simulink model "SS_1029"  (R2014a)
settings: Solver=FixedStepDiscrete  StartTime=0.0  StopTime=5  FixedStep=0.0005  RelTol=1e-3
values from neighbouring files (symbols this model uses):
  APS_High_null = ecucoder_cal(APS_High_null)    [SS.m]
  APS_High_x = ecucoder_cal(APS_High_x)    [SS.m]
  APS_High_y = ecucoder_cal(APS_High_y)    [SS.m]
  APS_Low_null = ecucoder_cal(APS_Low_null)    [SS.m]
  APS_low_x = ecucoder_cal(APS_low_x)    [SS.m]
  APS_low_y = ecucoder_cal(APS_low_y)    [SS.m]
  BrakeSignal_cal = ecucoder_cal(BrakeSignal_cal)    [SS.m]
  CustomReduceFactor_cal = ecucoder_cal(CustomReduceFactor_cal)    [SS.m]
  Differential_cal = ecucoder_cal(Differential_cal)    [SS.m]
  LowSOCWarning_cal = ecucoder_cal(LowSOCWarning_cal)    [SS.m]
  MotorTemperatureHigh_cal = ecucoder_cal(MotorTemperatureHigh_cal)    [SS.m]
  MotorTemperatureLow_cal = ecucoder_cal(MotorTemperatureLow_cal)    [SS.m]
  OilPressure_x = ecucoder_cal(OilPressure_x)    [SS.m]
  OilPressure_y = ecucoder_cal(OilPressure_y)    [SS.m]
  PowerBias_cal = ecucoder_cal(PowerBias_cal)    [SS.m]
  SpeedLimitFactor_x = ecucoder_cal(SpeedLimitFactor_x)    [SS.m]
  SpeedLimitFactor_y = ecucoder_cal(SpeedLimitFactor_y)    [SS.m]
  TorqueLimitNegativ_cal = ecucoder_cal(TorqueLimitNegativ_cal)    [SS.m]
  TorqueLimitPositiv_cal = ecucoder_cal(TorqueLimitPositiv_cal)    [SS.m]
libraries: simulink x101, ec55xxlib x31
(part 2 of 3)

== system SS_1029/HardWare_Input/In1_Message/Function-Call Subsystem1 ==
  Enable : Inport
  CANMsg : Inport  Port=2
  function : TriggerPort  TriggerType=function-call
  Subsystem : Subsystem
  AMK_TempMotor : Outport
  AMK_TempInverter : Outport  Port=2
  wires:
  CANMsg/1 -> Subsystem/1(In1)
  Subsystem/1(AMK_TempMotor) -> AMK_TempMotor/1
  Subsystem/2(AMK_TempInverter) -> AMK_TempInverter/1
  Enable/1 -> Subsystem/Enable

== system SS_1029/HardWare_Input/In2_Message/Function-Call Subsystem ==
  Enable : Inport
  CANMsg : Inport  Port=2
  function : TriggerPort  TriggerType=function-call
  Subsystem1 : Subsystem
  AMK_ActuralVelocity : Outport
  AMK_ActuralTorque : Outport  Port=2
  AMK_bSystemReady : Outport  Port=3
  AMK_bError : Outport  Port=4
  AMK_bQuitDcOn : Outport  Port=5
  "AMK_bQuitInverterOn " : Outport  Port=6
  wires:
  CANMsg/1 -> Subsystem1/1(In1)
  Subsystem1/1(Out1) -> AMK_bSystemReady/1
  Subsystem1/2(Out2) -> AMK_bError/1
  Subsystem1/3(Out3) -> AMK_bQuitDcOn/1
  Subsystem1/4(Out4) -> "AMK_bQuitInverterOn "/1
  Subsystem1/5(Out5) -> AMK_ActuralVelocity/1
  Subsystem1/6(Out6) -> AMK_ActuralTorque/1
  Enable/1 -> Subsystem1/Enable

== system SS_1029/HardWare_Input/In2_Message/Function-Call Subsystem1 ==
  Enable : Inport
  CANMsg : Inport  Port=2
  function : TriggerPort  TriggerType=function-call
  Subsystem : Subsystem
  AMK_TempMotor : Outport
  AMK_TempInverter : Outport  Port=2
  wires:
  CANMsg/1 -> Subsystem/1(In1)
  Subsystem/1(AMK_TempMotor) -> AMK_TempMotor/1
  Subsystem/2(AMK_TempInverter) -> AMK_TempInverter/1
  Enable/1 -> Subsystem/Enable

== system SS_1029/HardWare_Input/In3_Message/Function-Call Subsystem ==
  Enable : Inport
  CANMsg : Inport  Port=2
  function : TriggerPort  TriggerType=function-call
  Subsystem1 : Subsystem
  AMK_ActuralVelocity : Outport
  AMK_ActuralTorque : Outport  Port=2
  AMK_bSystemReady : Outport  Port=3
  AMK_bError : Outport  Port=4
  AMK_bQuitDcOn : Outport  Port=5
  "AMK_bQuitInverterOn " : Outport  Port=6
  wires:
  CANMsg/1 -> Subsystem1/1(In1)
  Subsystem1/1(Out1) -> AMK_bSystemReady/1
  Subsystem1/2(Out2) -> AMK_bError/1
  Subsystem1/3(Out3) -> AMK_bQuitDcOn/1
  Subsystem1/4(Out4) -> "AMK_bQuitInverterOn "/1
  Subsystem1/5(Out5) -> AMK_ActuralVelocity/1
  Subsystem1/6(Out6) -> AMK_ActuralTorque/1
  Enable/1 -> Subsystem1/Enable

== system SS_1029/HardWare_Input/In3_Message/Function-Call Subsystem1 ==
  Enable : Inport
  CANMsg : Inport  Port=2
  function : TriggerPort  TriggerType=function-call
  Subsystem : Subsystem
  AMK_TempMotor : Outport
  AMK_TempInverter : Outport  Port=2
  wires:
  CANMsg/1 -> Subsystem/1(In1)
  Subsystem/1(AMK_TempMotor) -> AMK_TempMotor/1
  Subsystem/2(AMK_TempInverter) -> AMK_TempInverter/1
  Enable/1 -> Subsystem/Enable

== system SS_1029/HardWare_Input/In4_Message/Function-Call Subsystem ==
  Enable : Inport
  CANMsg : Inport  Port=2
  function : TriggerPort  TriggerType=function-call
  Subsystem1 : Subsystem
  AMK_ActuralVelocity : Outport
  AMK_ActuralTorque : Outport  Port=2
  AMK_bSystemReady : Outport  Port=3
  AMK_bError : Outport  Port=4
  AMK_bQuitDcOn : Outport  Port=5
  "AMK_bQuitInverterOn " : Outport  Port=6
  wires:
  CANMsg/1 -> Subsystem1/1(In1)
  Subsystem1/1(Out1) -> AMK_bSystemReady/1
  Subsystem1/2(Out2) -> AMK_bError/1
  Subsystem1/3(Out3) -> AMK_bQuitDcOn/1
  Subsystem1/4(Out4) -> "AMK_bQuitInverterOn "/1
  Subsystem1/5(Out5) -> AMK_ActuralVelocity/1
  Subsystem1/6(Out6) -> AMK_ActuralTorque/1
  Enable/1 -> Subsystem1/Enable

== system SS_1029/HardWare_Input/In4_Message/Function-Call Subsystem1 ==
  Enable : Inport
  CANMsg : Inport  Port=2
  function : TriggerPort  TriggerType=function-call
  Subsystem : Subsystem
  AMK_TempMotor : Outport
  AMK_TempInverter : Outport  Port=2
  wires:
  CANMsg/1 -> Subsystem/1(In1)
  Subsystem/1(AMK_TempMotor) -> AMK_TempMotor/1
  Subsystem/2(AMK_TempInverter) -> AMK_TempInverter/1
  Enable/1 -> Subsystem/Enable

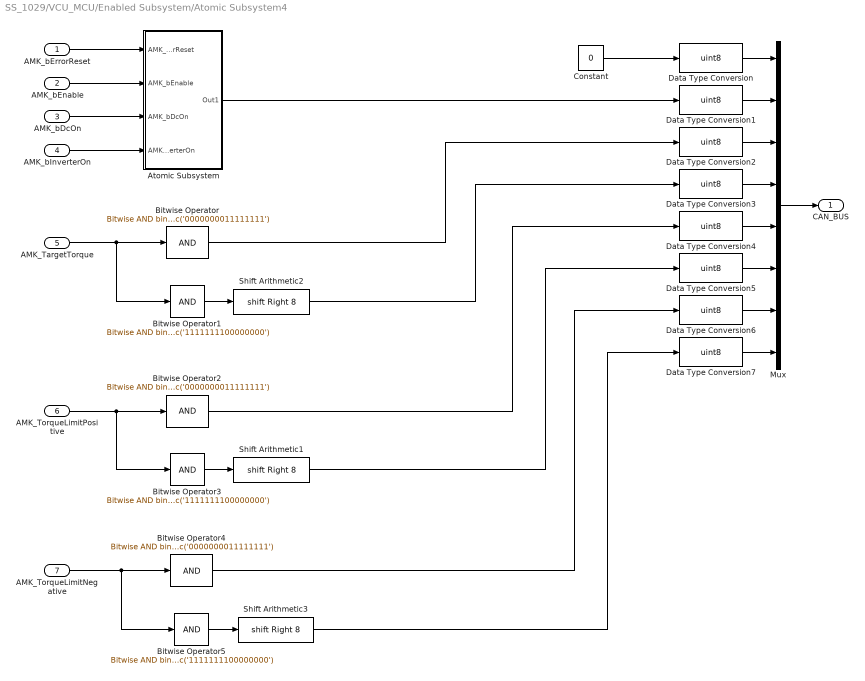
== system SS_1029/VCU_MCU/Enabled Subsystem/Atomic Subsystem4 ==
  AMK_bErrorReset : Inport
  AMK_bEnable : Inport  Port=2
  AMK_bDcOn : Inport  Port=3
  AMK_bInverterOn : Inport  Port=4
  AMK_TargetTorque : Inport  Port=5
  AMK_TorqueLimitPositive : Inport  Port=6
  AMK_TorqueLimitNegative : Inport  Port=7
  Atomic Subsystem : Subsystem  TreatAsAtomicUnit=on
  Bitwise Operator : simulink/Logic and Bit Operations/Bitwise Operator  logicop=AND  UseBitMask=on  BitMask=bin2dec('0000000011111111')  BitMaskRealWorld=Stored Integer
  Bitwise Operator1 : simulink/Logic and Bit Operations/Bitwise Operator  logicop=AND  UseBitMask=on  BitMask=bin2dec('1111111100000000')  BitMaskRealWorld=Stored Integer
  Bitwise Operator2 : simulink/Logic and Bit Operations/Bitwise Operator  logicop=AND  UseBitMask=on  BitMask=bin2dec('0000000011111111')  BitMaskRealWorld=Stored Integer
  Bitwise Operator3 : simulink/Logic and Bit Operations/Bitwise Operator  logicop=AND  UseBitMask=on  BitMask=bin2dec('1111111100000000')  BitMaskRealWorld=Stored Integer
  Bitwise Operator4 : simulink/Logic and Bit Operations/Bitwise Operator  logicop=AND  UseBitMask=on  BitMask=bin2dec('0000000011111111')  BitMaskRealWorld=Stored Integer
  Bitwise Operator5 : simulink/Logic and Bit Operations/Bitwise Operator  logicop=AND  UseBitMask=on  BitMask=bin2dec('1111111100000000')  BitMaskRealWorld=Stored Integer
  Constant : Constant  Value=0  OutDataTypeStr=uint8  SampleTime=-1
  Data Type Conversion{,1..7} (8 alike) : DataTypeConversion  OutDataTypeStr=uint8
  Mux : Mux  Inputs=8
  Shift Arithmetic1 : ArithShift  BitShiftNumber=8  BitShiftDirection=Right
  Shift Arithmetic2 : ArithShift  BitShiftNumber=8  BitShiftDirection=Right
  Shift Arithmetic3 : ArithShift  BitShiftNumber=8  BitShiftDirection=Right
  CAN_BUS : Outport
  wires:
  Mux/1 -> CAN_BUS/1
  Data Type Conversion/1 -> Mux/1
  Data Type Conversion1/1 -> Mux/2
  Data Type Conversion2/1 -> Mux/3
  Data Type Conversion3/1 -> Mux/4
  Data Type Conversion4/1 -> Mux/5
  Data Type Conversion5/1 -> Mux/6
  Data Type Conversion6/1 -> Mux/7
  Data Type Conversion7/1 -> Mux/8
  Constant/1 -> Data Type Conversion/1
  AMK_bErrorReset/1 -> Atomic Subsystem/1(AMK_bErrorReset)
  AMK_bEnable/1 -> Atomic Subsystem/2(AMK_bEnable)
  AMK_bDcOn/1 -> Atomic Subsystem/3(AMK_bDcOn)
  AMK_bInverterOn/1 -> Atomic Subsystem/4(AMK_bInverterOn)
  Atomic Subsystem/1(Out1) -> Data Type Conversion1/1
  AMK_TargetTorque/1 -> Bitwise Operator1/1, Bitwise Operator/1
  Bitwise Operator/1 -> Data Type Conversion2/1
  Bitwise Operator1/1 -> Shift Arithmetic2/1
  Shift Arithmetic2/1 -> Data Type Conversion3/1
  AMK_TorqueLimitPositive/1 -> Bitwise Operator3/1, Bitwise Operator2/1
  Bitwise Operator3/1 -> Shift Arithmetic1/1
  Bitwise Operator2/1 -> Data Type Conversion4/1
  Shift Arithmetic1/1 -> Data Type Conversion5/1
  AMK_TorqueLimitNegative/1 -> Bitwise Operator5/1, Bitwise Operator4/1
  Bitwise Operator5/1 -> Shift Arithmetic3/1
  Bitwise Operator4/1 -> Data Type Conversion6/1
  Shift Arithmetic3/1 -> Data Type Conversion7/1

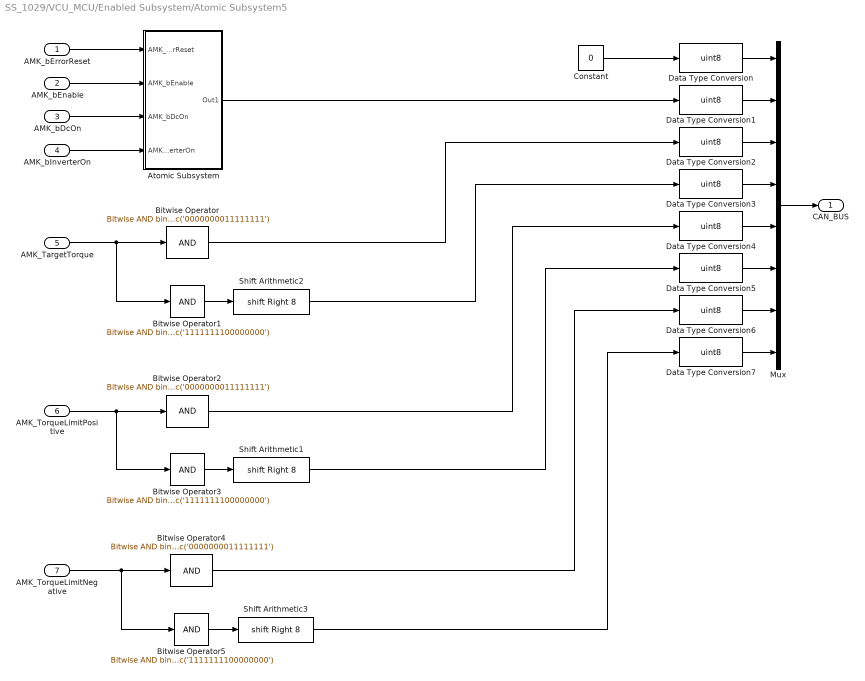
== system SS_1029/VCU_MCU/Enabled Subsystem/Atomic Subsystem5 ==
  AMK_bErrorReset : Inport
  AMK_bEnable : Inport  Port=2
  AMK_bDcOn : Inport  Port=3
  AMK_bInverterOn : Inport  Port=4
  AMK_TargetTorque : Inport  Port=5
  AMK_TorqueLimitPositive : Inport  Port=6
  AMK_TorqueLimitNegative : Inport  Port=7
  Atomic Subsystem : Subsystem  TreatAsAtomicUnit=on
  Bitwise Operator : simulink/Logic and Bit Operations/Bitwise Operator  logicop=AND  UseBitMask=on  BitMask=bin2dec('0000000011111111')  BitMaskRealWorld=Stored Integer
  Bitwise Operator1 : simulink/Logic and Bit Operations/Bitwise Operator  logicop=AND  UseBitMask=on  BitMask=bin2dec('1111111100000000')  BitMaskRealWorld=Stored Integer
  Bitwise Operator2 : simulink/Logic and Bit Operations/Bitwise Operator  logicop=AND  UseBitMask=on  BitMask=bin2dec('0000000011111111')  BitMaskRealWorld=Stored Integer
  Bitwise Operator3 : simulink/Logic and Bit Operations/Bitwise Operator  logicop=AND  UseBitMask=on  BitMask=bin2dec('1111111100000000')  BitMaskRealWorld=Stored Integer
  Bitwise Operator4 : simulink/Logic and Bit Operations/Bitwise Operator  logicop=AND  UseBitMask=on  BitMask=bin2dec('0000000011111111')  BitMaskRealWorld=Stored Integer
  Bitwise Operator5 : simulink/Logic and Bit Operations/Bitwise Operator  logicop=AND  UseBitMask=on  BitMask=bin2dec('1111111100000000')  BitMaskRealWorld=Stored Integer
  Constant : Constant  Value=0  OutDataTypeStr=uint8  SampleTime=-1
  Data Type Conversion{,1..7} (8 alike) : DataTypeConversion  OutDataTypeStr=uint8
  Mux : Mux  Inputs=8
  Shift Arithmetic1 : ArithShift  BitShiftNumber=8  BitShiftDirection=Right
  Shift Arithmetic2 : ArithShift  BitShiftNumber=8  BitShiftDirection=Right
  Shift Arithmetic3 : ArithShift  BitShiftNumber=8  BitShiftDirection=Right
  CAN_BUS : Outport
  wires:
  Mux/1 -> CAN_BUS/1
  Data Type Conversion/1 -> Mux/1
  Data Type Conversion1/1 -> Mux/2
  Data Type Conversion2/1 -> Mux/3
  Data Type Conversion3/1 -> Mux/4
  Data Type Conversion4/1 -> Mux/5
  Data Type Conversion5/1 -> Mux/6
  Data Type Conversion6/1 -> Mux/7
  Data Type Conversion7/1 -> Mux/8
  Constant/1 -> Data Type Conversion/1
  AMK_bErrorReset/1 -> Atomic Subsystem/1(AMK_bErrorReset)
  AMK_bEnable/1 -> Atomic Subsystem/2(AMK_bEnable)
  AMK_bDcOn/1 -> Atomic Subsystem/3(AMK_bDcOn)
  AMK_bInverterOn/1 -> Atomic Subsystem/4(AMK_bInverterOn)
  Atomic Subsystem/1(Out1) -> Data Type Conversion1/1
  AMK_TargetTorque/1 -> Bitwise Operator1/1, Bitwise Operator/1
  Bitwise Operator/1 -> Data Type Conversion2/1
  Bitwise Operator1/1 -> Shift Arithmetic2/1
  Shift Arithmetic2/1 -> Data Type Conversion3/1
  AMK_TorqueLimitPositive/1 -> Bitwise Operator3/1, Bitwise Operator2/1
  Bitwise Operator3/1 -> Shift Arithmetic1/1
  Bitwise Operator2/1 -> Data Type Conversion4/1
  Shift Arithmetic1/1 -> Data Type Conversion5/1
  AMK_TorqueLimitNegative/1 -> Bitwise Operator5/1, Bitwise Operator4/1
  Bitwise Operator5/1 -> Shift Arithmetic3/1
  Bitwise Operator4/1 -> Data Type Conversion6/1
  Shift Arithmetic3/1 -> Data Type Conversion7/1

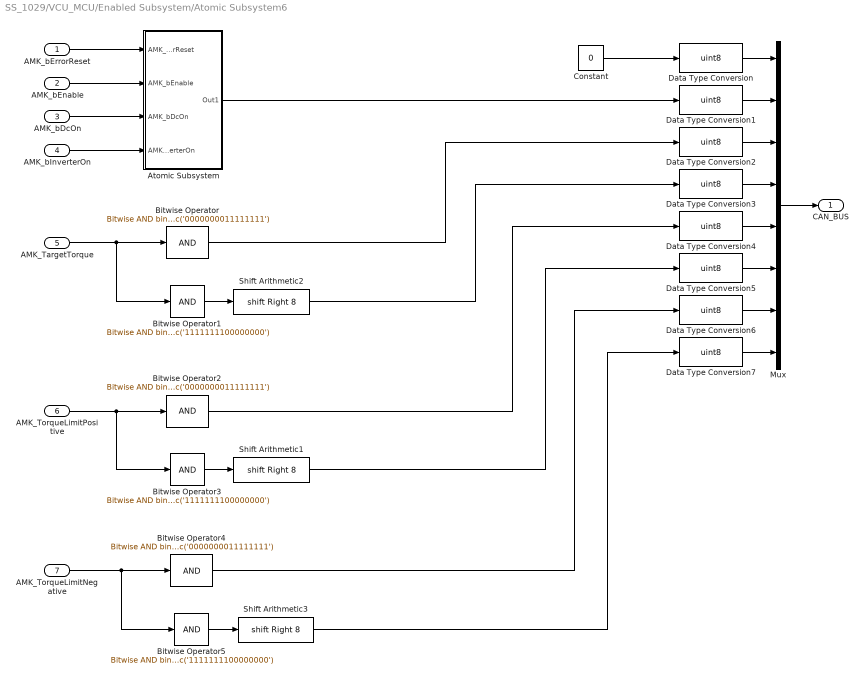
== system SS_1029/VCU_MCU/Enabled Subsystem/Atomic Subsystem6 ==
  AMK_bErrorReset : Inport
  AMK_bEnable : Inport  Port=2
  AMK_bDcOn : Inport  Port=3
  AMK_bInverterOn : Inport  Port=4
  AMK_TargetTorque : Inport  Port=5
  AMK_TorqueLimitPositive : Inport  Port=6
  AMK_TorqueLimitNegative : Inport  Port=7
  Atomic Subsystem : Subsystem  TreatAsAtomicUnit=on
  Bitwise Operator : simulink/Logic and Bit Operations/Bitwise Operator  logicop=AND  UseBitMask=on  BitMask=bin2dec('0000000011111111')  BitMaskRealWorld=Stored Integer
  Bitwise Operator1 : simulink/Logic and Bit Operations/Bitwise Operator  logicop=AND  UseBitMask=on  BitMask=bin2dec('1111111100000000')  BitMaskRealWorld=Stored Integer
  Bitwise Operator2 : simulink/Logic and Bit Operations/Bitwise Operator  logicop=AND  UseBitMask=on  BitMask=bin2dec('0000000011111111')  BitMaskRealWorld=Stored Integer
  Bitwise Operator3 : simulink/Logic and Bit Operations/Bitwise Operator  logicop=AND  UseBitMask=on  BitMask=bin2dec('1111111100000000')  BitMaskRealWorld=Stored Integer
  Bitwise Operator4 : simulink/Logic and Bit Operations/Bitwise Operator  logicop=AND  UseBitMask=on  BitMask=bin2dec('0000000011111111')  BitMaskRealWorld=Stored Integer
  Bitwise Operator5 : simulink/Logic and Bit Operations/Bitwise Operator  logicop=AND  UseBitMask=on  BitMask=bin2dec('1111111100000000')  BitMaskRealWorld=Stored Integer
  Constant : Constant  Value=0  OutDataTypeStr=uint8  SampleTime=-1
  Data Type Conversion{,1..7} (8 alike) : DataTypeConversion  OutDataTypeStr=uint8
  Mux : Mux  Inputs=8
  Shift Arithmetic1 : ArithShift  BitShiftNumber=8  BitShiftDirection=Right
  Shift Arithmetic2 : ArithShift  BitShiftNumber=8  BitShiftDirection=Right
  Shift Arithmetic3 : ArithShift  BitShiftNumber=8  BitShiftDirection=Right
  CAN_BUS : Outport
  wires:
  Mux/1 -> CAN_BUS/1
  Data Type Conversion/1 -> Mux/1
  Data Type Conversion1/1 -> Mux/2
  Data Type Conversion2/1 -> Mux/3
  Data Type Conversion3/1 -> Mux/4
  Data Type Conversion4/1 -> Mux/5
  Data Type Conversion5/1 -> Mux/6
  Data Type Conversion6/1 -> Mux/7
  Data Type Conversion7/1 -> Mux/8
  Constant/1 -> Data Type Conversion/1
  AMK_bErrorReset/1 -> Atomic Subsystem/1(AMK_bErrorReset)
  AMK_bEnable/1 -> Atomic Subsystem/2(AMK_bEnable)
  AMK_bDcOn/1 -> Atomic Subsystem/3(AMK_bDcOn)
  AMK_bInverterOn/1 -> Atomic Subsystem/4(AMK_bInverterOn)
  Atomic Subsystem/1(Out1) -> Data Type Conversion1/1
  AMK_TargetTorque/1 -> Bitwise Operator1/1, Bitwise Operator/1
  Bitwise Operator/1 -> Data Type Conversion2/1
  Bitwise Operator1/1 -> Shift Arithmetic2/1
  Shift Arithmetic2/1 -> Data Type Conversion3/1
  AMK_TorqueLimitPositive/1 -> Bitwise Operator3/1, Bitwise Operator2/1
  Bitwise Operator3/1 -> Shift Arithmetic1/1
  Bitwise Operator2/1 -> Data Type Conversion4/1
  Shift Arithmetic1/1 -> Data Type Conversion5/1
  AMK_TorqueLimitNegative/1 -> Bitwise Operator5/1, Bitwise Operator4/1
  Bitwise Operator5/1 -> Shift Arithmetic3/1
  Bitwise Operator4/1 -> Data Type Conversion6/1
  Shift Arithmetic3/1 -> Data Type Conversion7/1

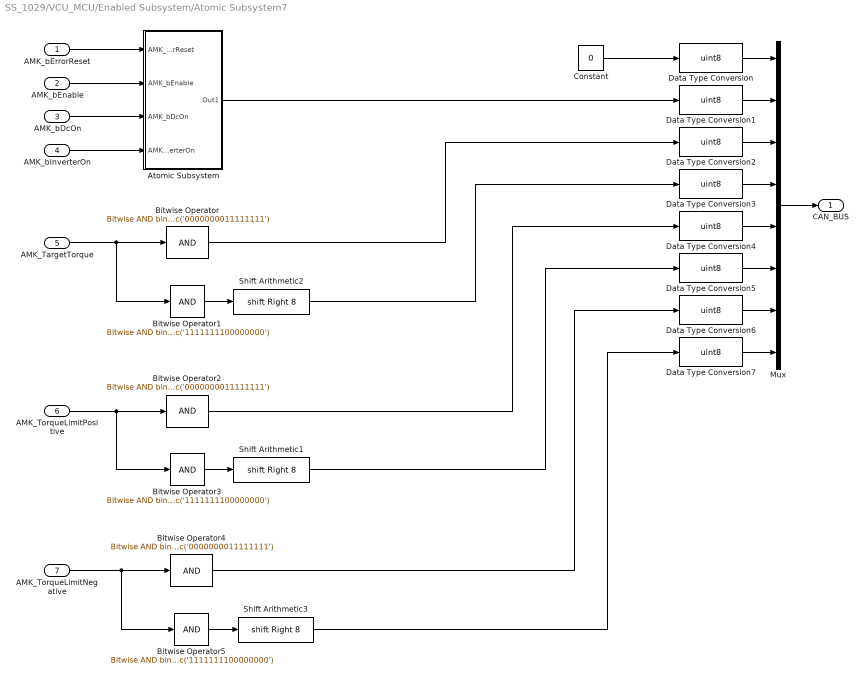
== system SS_1029/VCU_MCU/Enabled Subsystem/Atomic Subsystem7 ==
  AMK_bErrorReset : Inport
  AMK_bEnable : Inport  Port=2
  AMK_bDcOn : Inport  Port=3
  AMK_bInverterOn : Inport  Port=4
  AMK_TargetTorque : Inport  Port=5
  AMK_TorqueLimitPositive : Inport  Port=6
  AMK_TorqueLimitNegative : Inport  Port=7
  Atomic Subsystem : Subsystem  TreatAsAtomicUnit=on
  Bitwise Operator : simulink/Logic and Bit Operations/Bitwise Operator  logicop=AND  UseBitMask=on  BitMask=bin2dec('0000000011111111')  BitMaskRealWorld=Stored Integer
  Bitwise Operator1 : simulink/Logic and Bit Operations/Bitwise Operator  logicop=AND  UseBitMask=on  BitMask=bin2dec('1111111100000000')  BitMaskRealWorld=Stored Integer
  Bitwise Operator2 : simulink/Logic and Bit Operations/Bitwise Operator  logicop=AND  UseBitMask=on  BitMask=bin2dec('0000000011111111')  BitMaskRealWorld=Stored Integer
  Bitwise Operator3 : simulink/Logic and Bit Operations/Bitwise Operator  logicop=AND  UseBitMask=on  BitMask=bin2dec('1111111100000000')  BitMaskRealWorld=Stored Integer
  Bitwise Operator4 : simulink/Logic and Bit Operations/Bitwise Operator  logicop=AND  UseBitMask=on  BitMask=bin2dec('0000000011111111')  BitMaskRealWorld=Stored Integer
  Bitwise Operator5 : simulink/Logic and Bit Operations/Bitwise Operator  logicop=AND  UseBitMask=on  BitMask=bin2dec('1111111100000000')  BitMaskRealWorld=Stored Integer
  Constant : Constant  Value=0  OutDataTypeStr=uint8  SampleTime=-1
  Data Type Conversion{,1..7} (8 alike) : DataTypeConversion  OutDataTypeStr=uint8
  Mux : Mux  Inputs=8
  Shift Arithmetic1 : ArithShift  BitShiftNumber=8  BitShiftDirection=Right
  Shift Arithmetic2 : ArithShift  BitShiftNumber=8  BitShiftDirection=Right
  Shift Arithmetic3 : ArithShift  BitShiftNumber=8  BitShiftDirection=Right
  CAN_BUS : Outport
  wires:
  Mux/1 -> CAN_BUS/1
  Data Type Conversion/1 -> Mux/1
  Data Type Conversion1/1 -> Mux/2
  Data Type Conversion2/1 -> Mux/3
  Data Type Conversion3/1 -> Mux/4
  Data Type Conversion4/1 -> Mux/5
  Data Type Conversion5/1 -> Mux/6
  Data Type Conversion6/1 -> Mux/7
  Data Type Conversion7/1 -> Mux/8
  Constant/1 -> Data Type Conversion/1
  AMK_bErrorReset/1 -> Atomic Subsystem/1(AMK_bErrorReset)
  AMK_bEnable/1 -> Atomic Subsystem/2(AMK_bEnable)
  AMK_bDcOn/1 -> Atomic Subsystem/3(AMK_bDcOn)
  AMK_bInverterOn/1 -> Atomic Subsystem/4(AMK_bInverterOn)
  Atomic Subsystem/1(Out1) -> Data Type Conversion1/1
  AMK_TargetTorque/1 -> Bitwise Operator1/1, Bitwise Operator/1
  Bitwise Operator/1 -> Data Type Conversion2/1
  Bitwise Operator1/1 -> Shift Arithmetic2/1
  Shift Arithmetic2/1 -> Data Type Conversion3/1
  AMK_TorqueLimitPositive/1 -> Bitwise Operator3/1, Bitwise Operator2/1
  Bitwise Operator3/1 -> Shift Arithmetic1/1
  Bitwise Operator2/1 -> Data Type Conversion4/1
  Shift Arithmetic1/1 -> Data Type Conversion5/1
  AMK_TorqueLimitNegative/1 -> Bitwise Operator5/1, Bitwise Operator4/1
  Bitwise Operator5/1 -> Shift Arithmetic3/1
  Bitwise Operator4/1 -> Data Type Conversion6/1
  Shift Arithmetic3/1 -> Data Type Conversion7/1

== system SS_1029/VCU_MCU/Enabled Subsystem/Atomic Subsystem8 ==
  Logicvalue : Inport
  PowerReduceFactor : Inport  Port=2
  SOCReduceFactor : Inport  Port=3
  Powersum : Inport  Port=4
  Bitwise Operator : simulink/Logic and Bit Operations/Bitwise Operator  logicop=AND  UseBitMask=on  BitMask=bin2dec('0000000011111111')  BitMaskRealWorld=Stored Integer
  Bitwise Operator1 : simulink/Logic and Bit Operations/Bitwise Operator  logicop=AND  UseBitMask=on  BitMask=bin2dec('1111111100000000')  BitMaskRealWorld=Stored Integer
  Constant : Constant  Value=0  SampleTime=-1
  Constant1 : Constant  Value=0  SampleTime=-1
  Constant2 : Constant  Value=0  SampleTime=-1
  Data Type Conversion{,1..2,4..8} (8 alike) : DataTypeConversion  OutDataTypeStr=uint8
  Data Type Conversion3 : DataTypeConversion  OutDataTypeStr=uint16
  Gain{,1..3} (4 alike) : Gain  Gain=100
  Mux : Mux  Inputs=8
  Shift Arithmetic1 : ArithShift  BitShiftNumber=8  BitShiftDirection=Right
  Out1 : Outport
  wires:
  Logicvalue/1 -> Gain/1
  PowerReduceFactor/1 -> Gain1/1
  SOCReduceFactor/1 -> Gain2/1
  Powersum/1 -> Gain3/1
  Gain/1 -> Data Type Conversion/1
  Gain1/1 -> Data Type Conversion1/1
  Gain2/1 -> Data Type Conversion2/1
  Gain3/1 -> Data Type Conversion3/1
  Data Type Conversion/1 -> Mux/1
  Data Type Conversion1/1 -> Mux/2
  Data Type Conversion2/1 -> Mux/3
  Data Type Conversion3/1 -> Bitwise Operator/1, Bitwise Operator1/1
  Bitwise Operator1/1 -> Shift Arithmetic1/1
  Shift Arithmetic1/1 -> Data Type Conversion4/1
  Bitwise Operator/1 -> Data Type Conversion5/1
  Data Type Conversion5/1 -> Mux/5
  Data Type Conversion4/1 -> Mux/4
  Constant/1 -> Data Type Conversion6/1
  Data Type Conversion6/1 -> Mux/6
  Constant1/1 -> Data Type Conversion7/1
  Data Type Conversion7/1 -> Mux/7
  Constant2/1 -> Data Type Conversion8/1
  Data Type Conversion8/1 -> Mux/8
  Mux/1 -> Out1/1

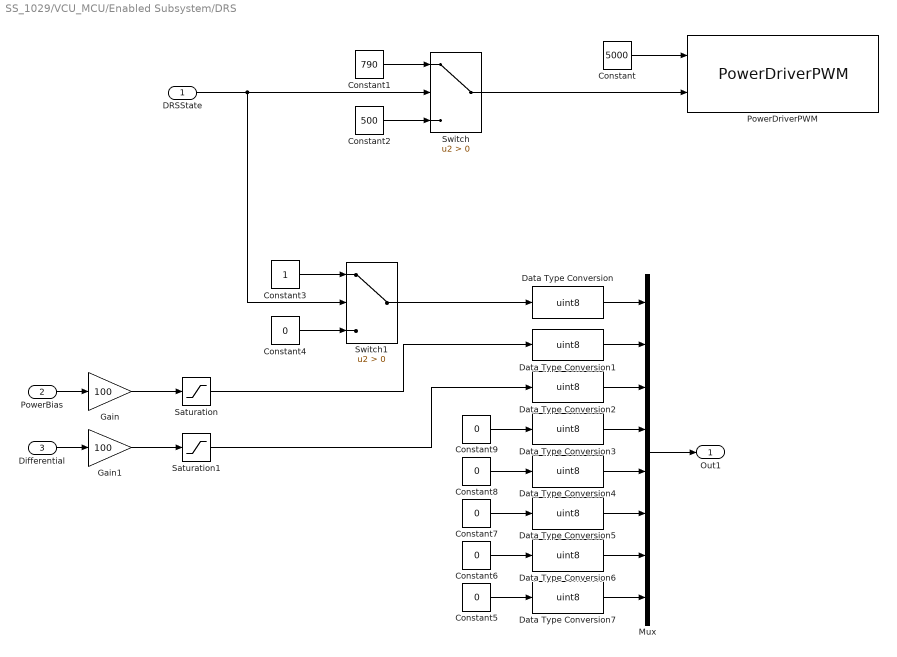
== system SS_1029/VCU_MCU/Enabled Subsystem/DRS ==
  DRSState : Inport
  PowerBias : Inport  Port=2
  "Differential " : Inport  Port=3
  Constant : Constant  Value=5000  OutDataTypeStr=uint32  SampleTime=-1
  Constant1 : Constant  Value=790  OutDataTypeStr=uint32  SampleTime=-1
  Constant2 : Constant  Value=500  OutDataTypeStr=uint32  SampleTime=-1
  Constant3 : Constant  OutDataTypeStr=uint8  SampleTime=-1
  Constant{4..9} (6 alike) : Constant  Value=0  OutDataTypeStr=uint8  SampleTime=-1
  Data Type Conversion{,1..7} (8 alike) : DataTypeConversion  OutDataTypeStr=uint8
  Gain : Gain  Gain=100
  Gain1 : Gain  Gain=100
  Mux : Mux  Inputs=8
  PowerDriverPWM : ec55xxlib/RapidECU_U2/06PowerDriverPWM/PowerDriverPWM  channel=118: O_PWM12_HS2A9  sampletime=-1
  Saturation : Saturate  UpperLimit=100  LowerLimit=0
  Saturation1 : Saturate  UpperLimit=100  LowerLimit=0
  Switch : Switch  Criteria=u2 > Threshold
  Switch1 : Switch  Criteria=u2 > Threshold
  Out1 : Outport
  wires:
  DRSState/1 -> Switch1/2, Switch/2
  Constant/1 -> PowerDriverPWM/1
  Switch/1 -> PowerDriverPWM/2
  Constant1/1 -> Switch/1
  Constant2/1 -> Switch/3
  Constant4/1 -> Switch1/3
  Constant3/1 -> Switch1/1
  Switch1/1 -> Data Type Conversion/1
  Data Type Conversion/1 -> Mux/1
  Data Type Conversion1/1 -> Mux/2
  Data Type Conversion2/1 -> Mux/3
  Data Type Conversion3/1 -> Mux/4
  Data Type Conversion4/1 -> Mux/5
  Data Type Conversion5/1 -> Mux/6
  Data Type Conversion6/1 -> Mux/7
  Data Type Conversion7/1 -> Mux/8
  Constant5/1 -> Data Type Conversion7/1
  Constant6/1 -> Data Type Conversion6/1
  Constant7/1 -> Data Type Conversion5/1
  Constant8/1 -> Data Type Conversion4/1
  Constant9/1 -> Data Type Conversion3/1
  Mux/1 -> Out1/1
  "Differential "/1 -> Gain1/1
  PowerBias/1 -> Gain/1
  Gain1/1 -> Saturation1/1
  Gain/1 -> Saturation/1
  Saturation/1 -> Data Type Conversion1/1
  Saturation1/1 -> Data Type Conversion2/1

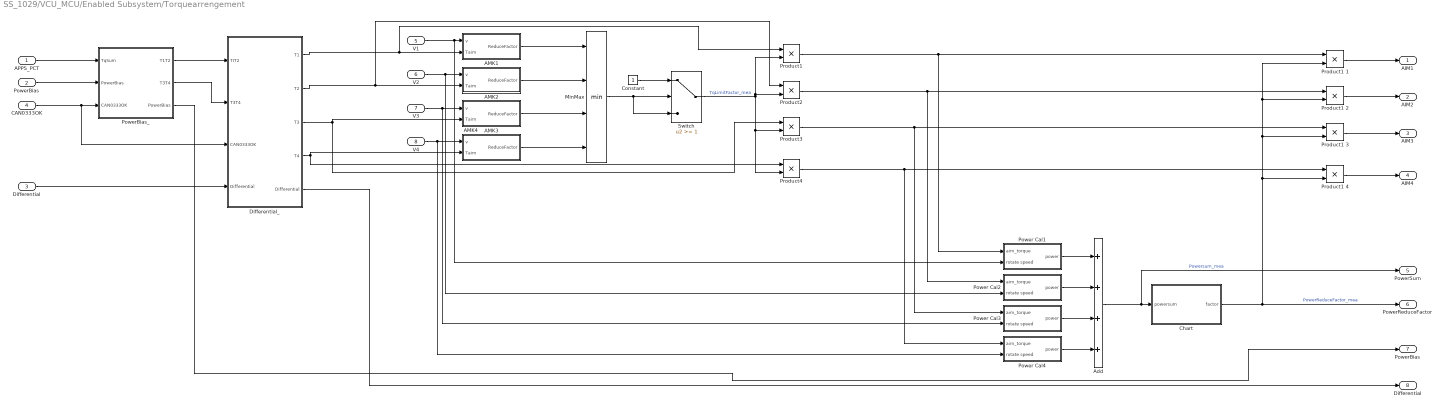
== system SS_1029/VCU_MCU/Enabled Subsystem/Torquearrengement ==
  APPS_PCT : Inport
  PowerBias : Inport  Port=2
  Differential : Inport  Port=3
  CAN0333OK : Inport  Port=4
  V1 : Inport  Port=5
  V2 : Inport  Port=6
  V3 : Inport  Port=7
  V4 : Inport  Port=8
  AMK1 : Subsystem  TreatAsAtomicUnit=on
  AMK2 : Subsystem  TreatAsAtomicUnit=on
  AMK3 : Subsystem  TreatAsAtomicUnit=on
  AMK4 : Subsystem  TreatAsAtomicUnit=on
  Add : Sum  Inputs=++++
  Chart : Stateflow chart  TreatAsAtomicUnit=on
  Constant : Constant  OutDataTypeStr=single  SampleTime=-1
  Differential_ : Subsystem
  MinMax : MinMax  Inputs=4
  Power Cal1 : Subsystem  TreatAsAtomicUnit=on
  Power Cal2 : Subsystem  TreatAsAtomicUnit=on
  Power Cal3 : Subsystem  TreatAsAtomicUnit=on
  Power Cal4 : Subsystem  TreatAsAtomicUnit=on
  PowerBias_ : Subsystem  TreatAsAtomicUnit=on
  Product1 {,1..4} (5 alike) : Product
  Product2 : Product
  Product3 : Product
  "Product4 " : Product
  Switch : Switch  Threshold=1
  AIM1 : Outport
  AIM2 : Outport  Port=2
  AIM3 : Outport  Port=3
  AIM4 : Outport  Port=4
  PowerSum : Outport  Port=5
  PowerReduceFactor : Outport  Port=6
  "PowerBias " : Outport  Port=7
  "Differential " : Outport  Port=8
  wires:
  APPS_PCT/1 -> PowerBias_/1(TqSum)
  PowerBias_/1(T1T2) -> Differential_/1(TIT2)
  PowerBias_/2(T3T4) -> Differential_/2(T3T4)
  V4/1 -> Power Cal4/2("rotate speed "), AMK4/1(v)
  V3/1 -> Power Cal3/2("rotate speed "), AMK3/1(v)
  V2/1 -> AMK2/1(v), Power Cal2/2("rotate speed ")
  V1/1 -> Power Cal1/2("rotate speed "), AMK1/1(v)
  Differential_/1(T1) -> "Product1 "/1, AMK1/2(Taim)
  Differential_/2(T2) -> Product2/1, AMK2/2(Taim)
  Differential_/3(T3) -> Product3/1, AMK3/2(Taim)
  Differential_/4(T4) -> "Product4 "/1, AMK4/2(Taim)
  AMK1/1("ReduceFactor ") -> MinMax/1
  AMK2/1("ReduceFactor ") -> MinMax/2
  AMK3/1("ReduceFactor ") -> MinMax/3
  AMK4/1("ReduceFactor ") -> MinMax/4
  Constant/1 -> Switch/1
  MinMax/1 -> Switch/3, Switch/2
  "Product4 "/1 -> Product1 4/1, Power Cal4/1(aim_torque)
  Product3/1 -> Product1 3/1, Power Cal3/1(aim_torque)
  Product2/1 -> Product1 2/1, Power Cal2/1(aim_torque)
  "Product1 "/1 -> Product1 1/1, Power Cal1/1(aim_torque)
  Switch/1 -> "Product4 "/2, Product3/2, "Product1 "/2, Product2/2  "TqLimitFactor_mea"
  Add/1 -> PowerSum/1, Chart/1(powersum)  "Powersum_mea"
  Chart/1(factor) -> Product1 4/2, Product1 3/2, Product1 2/2, Product1 1/2, PowerReduceFactor/1  "PowerReduceFactor_mea"
  Power Cal1/1(power) -> Add/1
  Power Cal2/1(power) -> Add/2
  Power Cal3/1(power) -> Add/3
  Power Cal4/1(power) -> Add/4
  Product1 1/1 -> AIM1/1
  Product1 2/1 -> AIM2/1
  Product1 3/1 -> AIM3/1
  Product1 4/1 -> AIM4/1
  PowerBias/1 -> PowerBias_/2(PowerBias)
  CAN0333OK/1 -> Differential_/3(CAN0333OK), PowerBias_/3(CAN0333OK)
  Differential/1 -> Differential_/4(Differential)
  PowerBias_/3("PowerBias ") -> "PowerBias "/1
  Differential_/5("Differential ") -> "Differential "/1

== system SS_1029/VCU_MCU/Enabled Subsystem/speedlimit  ==
  v1 : Inport
  v2 : Inport  Port=2
  v3 : Inport  Port=3
  v4 : Inport  Port=4
  1-D Lookup Table : Lookup_n-D  NumberOfTableDimensions=1  BreakpointsForDimension1=SpeedLimitFactor_x  Table=SpeedLimitFactor_y  ExtrapMethod=Clip  InternalRulePriority=Speed  RndMeth=Simplest  InputSameDT=on
  D : Constant  Value=467.36  SampleTime=-1
  Divide : Product  Inputs=****//
  MinMax4 : MinMax  Inputs=4
  min2hour : Constant  Value=60  SampleTime=-1
  mm2km : Constant  Value=1000000  SampleTime=-1
  pi : Constant  Value=3.14  SampleTime=-1
  trans rate : Constant  Value=12.27  SampleTime=-1
  SpeedReduceFactor : Outport
  wires:
  1-D Lookup Table/1 -> SpeedReduceFactor/1
  v2/1 -> MinMax4/2
  v3/1 -> MinMax4/3
  v1/1 -> MinMax4/1
  mm2km/1 -> Divide/6
  min2hour/1 -> Divide/1
  Divide/1 -> 1-D Lookup Table/1
  pi/1 -> Divide/3
  MinMax4/1 -> Divide/4
  D/1 -> Divide/2
  trans rate/1 -> Divide/5
  v4/1 -> MinMax4/4

== system SS_1029/HardWare_Input/BMS Info/Subsystem/Subsystem ==
  CANMsg : Inport
  Enable : EnablePort
  Data Type Conversion1 : DataTypeConversion  OutDataTypeStr=uint8
  Data Type Conversion2 : DataTypeConversion  OutDataTypeStr=uint8
  Data Type Conversion3 : DataTypeConversion  OutDataTypeStr=uint8
  Demux : Demux  Outputs=8
  Terminator{4..8} (5 alike) : Terminator
  Voltage_MSB : Outport
  Voltage_LSB : Outport  Port=2
  SOC : Outport  Port=3
  wires:
  CANMsg/1 -> Demux/1
  Demux/1 -> Data Type Conversion3/1
  Demux/2 -> Data Type Conversion1/1
  Demux/3 -> Terminator4/1
  Demux/4 -> Terminator5/1
  Demux/6 -> Terminator6/1
  Data Type Conversion1/1 -> Voltage_LSB/1
  Demux/8 -> Terminator8/1
  Demux/5 -> Data Type Conversion2/1
  Demux/7 -> Terminator7/1
  Data Type Conversion3/1 -> Voltage_MSB/1
  Data Type Conversion2/1 -> SOC/1

== system SS_1029/HardWare_Input/DRS CMDInput/Subsystem/Subsystem ==
  CANMsg : Inport
  Enable : EnablePort
  Data Type Conversion{,1..4} (5 alike) : DataTypeConversion  OutDataTypeStr=uint8
  Demux : Demux  Outputs=8
  Gain : Gain  Gain=0.01  OutDataTypeStr=single
  Gain1 : Gain  Gain=0.01  OutDataTypeStr=single
  Saturation : Saturate  UpperLimit=100  LowerLimit=0  LinearizeAsGain=off
  Saturation1 : Saturate  UpperLimit=100  LowerLimit=0  LinearizeAsGain=off
  Terminator{6..10} (5 alike) : Terminator
  DRS : Outport
  PowerBias : Outport  Port=2
  Differential : Outport  Port=3
  wires:
  Demux/4 -> Terminator6/1
  Demux/8 -> Terminator10/1
  Demux/3 -> Data Type Conversion2/1
  Data Type Conversion/1 -> DRS/1
  CANMsg/1 -> Demux/1  "DRSCAN_MEA"
  Demux/2 -> Data Type Conversion1/1
  Demux/1 -> Data Type Conversion/1
  Demux/5 -> Terminator7/1
  Demux/6 -> Terminator8/1
  Demux/7 -> Terminator9/1
  Data Type Conversion1/1 -> Saturation/1
  Data Type Conversion2/1 -> Saturation1/1
  Saturation/1 -> Data Type Conversion3/1
  Saturation1/1 -> Data Type Conversion4/1
  Gain/1 -> PowerBias/1
  Gain1/1 -> Differential/1
  Data Type Conversion4/1 -> Gain1/1
  Data Type Conversion3/1 -> Gain/1

== system SS_1029/HardWare_Input/In1_Message/Function-Call Subsystem/Subsystem1 ==
  In1 : Inport
  Enable : EnablePort
  Add : Sum
  Add1 : Sum
  Data Type Conversion : DataTypeConversion  OutDataTypeStr=uint8
  Data Type Conversion{1..6} (6 alike) : DataTypeConversion  OutDataTypeStr=uint16
  Demux : Demux  Outputs=8
  Shift Arithmetic1 : ArithShift  BitShiftNumber=8  BitShiftDirection=Left
  Shift Arithmetic2 : ArithShift  BitShiftNumber=8  BitShiftDirection=Left
  Subsystem : Subsystem
  Terminator : Terminator
  Terminator1 : Terminator
  Terminator2 : Terminator
  Out1 : Outport
  Out2 : Outport  Port=2
  Out3 : Outport  Port=3
  Out4 : Outport  Port=4
  Out5 : Outport  Port=5
  Out6 : Outport  Port=6
  wires:
  In1/1 -> Demux/1
  Demux/1 -> Terminator/1
  Add1/1 -> Data Type Conversion6/1
  Data Type Conversion6/1 -> Out6/1
  Add/1 -> Data Type Conversion3/1
  Data Type Conversion/1 -> Subsystem/1(In1)
  Demux/3 -> Data Type Conversion1/1
  Demux/5 -> Data Type Conversion4/1
  Demux/6 -> Data Type Conversion5/1
  Demux/2 -> Data Type Conversion/1
  Demux/4 -> Data Type Conversion2/1
  Data Type Conversion2/1 -> Shift Arithmetic2/1
  Shift Arithmetic2/1 -> Add/2
  Data Type Conversion1/1 -> Add/1
  Data Type Conversion3/1 -> Out5/1
  Data Type Conversion5/1 -> Shift Arithmetic1/1
  Data Type Conversion4/1 -> Add1/1
  Shift Arithmetic1/1 -> Add1/2
  Subsystem/1(AMK_bSystemReady) -> Out1/1
  Subsystem/4(AMK_bQuitInverterOn) -> Out4/1
  Subsystem/3(AMK_bQuitDcOn) -> Out3/1
  Demux/7 -> Terminator1/1
  Subsystem/2(AMK_bError) -> Out2/1
  Demux/8 -> Terminator2/1

== system SS_1029/HardWare_Input/In1_Message/Function-Call Subsystem1/Subsystem ==
  In1 : Inport
  Enable : EnablePort
  Add1 : Sum
  Add2 : Sum
  Data Type Conversion1 : DataTypeConversion  OutDataTypeStr=single
  Data Type Conversion2 : DataTypeConversion  OutDataTypeStr=single
  Data Type Conversion{3..6} (4 alike) : DataTypeConversion  OutDataTypeStr=uint16
  Demux : Demux  Outputs=8
  Gain : Gain  Gain=0.1
  Gain1 : Gain  Gain=0.1
  Shift Arithmetic1 : ArithShift  BitShiftNumber=8  BitShiftDirection=Left
  Shift Arithmetic2 : ArithShift  BitShiftNumber=8  BitShiftDirection=Left
  Terminator{,1..3} (4 alike) : Terminator
  AMK_TempMotor : Outport
  AMK_TempInverter : Outport  Port=2
  wires:
  Data Type Conversion2/1 -> AMK_TempInverter/1
  Gain/1 -> Data Type Conversion1/1
  Add1/1 -> Gain/1
  Data Type Conversion1/1 -> AMK_TempMotor/1
  Data Type Conversion4/1 -> Add1/1
  Data Type Conversion5/1 -> Shift Arithmetic1/1
  Shift Arithmetic2/1 -> Add2/2
  Add2/1 -> Gain1/1
  Shift Arithmetic1/1 -> Add1/2
  Demux/2 -> Data Type Conversion5/1
  Gain1/1 -> Data Type Conversion2/1
  Demux/1 -> Data Type Conversion4/1
  Data Type Conversion3/1 -> Add2/1
  In1/1 -> Demux/1
  Data Type Conversion6/1 -> Shift Arithmetic2/1
  Demux/6 -> Terminator1/1
  Demux/5 -> Terminator/1
  Demux/4 -> Data Type Conversion6/1
  Demux/3 -> Data Type Conversion3/1
  Demux/8 -> Terminator3/1
  Demux/7 -> Terminator2/1

== system SS_1029/HardWare_Input/In2_Message/Function-Call Subsystem/Subsystem1 ==
  In1 : Inport
  Enable : EnablePort
  Add : Sum
  Add1 : Sum
  Data Type Conversion : DataTypeConversion  OutDataTypeStr=uint8
  Data Type Conversion{1..6} (6 alike) : DataTypeConversion  OutDataTypeStr=uint16
  Demux : Demux  Outputs=8
  Shift Arithmetic1 : ArithShift  BitShiftNumber=8  BitShiftDirection=Left
  Shift Arithmetic2 : ArithShift  BitShiftNumber=8  BitShiftDirection=Left
  Subsystem : Subsystem
  Terminator : Terminator
  Terminator1 : Terminator
  Terminator2 : Terminator
  Out1 : Outport
  Out2 : Outport  Port=2
  Out3 : Outport  Port=3
  Out4 : Outport  Port=4
  Out5 : Outport  Port=5
  Out6 : Outport  Port=6
  wires:
  In1/1 -> Demux/1
  Demux/1 -> Terminator/1
  Add1/1 -> Data Type Conversion6/1
  Data Type Conversion6/1 -> Out6/1
  Add/1 -> Data Type Conversion3/1
  Data Type Conversion/1 -> Subsystem/1(In1)
  Demux/3 -> Data Type Conversion1/1
  Demux/5 -> Data Type Conversion4/1
  Demux/6 -> Data Type Conversion5/1
  Demux/2 -> Data Type Conversion/1
  Demux/4 -> Data Type Conversion2/1
  Data Type Conversion2/1 -> Shift Arithmetic2/1
  Shift Arithmetic2/1 -> Add/2
  Data Type Conversion1/1 -> Add/1
  Data Type Conversion3/1 -> Out5/1
  Data Type Conversion5/1 -> Shift Arithmetic1/1
  Data Type Conversion4/1 -> Add1/1
  Shift Arithmetic1/1 -> Add1/2
  Subsystem/1(AMK_bSystemReady) -> Out1/1
  Subsystem/4(AMK_bQuitInverterOn) -> Out4/1
  Subsystem/3(AMK_bQuitDcOn) -> Out3/1
  Demux/7 -> Terminator1/1
  Subsystem/2(AMK_bError) -> Out2/1
  Demux/8 -> Terminator2/1

== system SS_1029/HardWare_Input/In2_Message/Function-Call Subsystem1/Subsystem ==
  In1 : Inport
  Enable : EnablePort
  Add1 : Sum
  Add2 : Sum
  Data Type Conversion1 : DataTypeConversion  OutDataTypeStr=single
  Data Type Conversion2 : DataTypeConversion  OutDataTypeStr=single
  Data Type Conversion{3..6} (4 alike) : DataTypeConversion  OutDataTypeStr=uint16
  Demux : Demux  Outputs=8
  Gain : Gain  Gain=0.1
  Gain1 : Gain  Gain=0.1
  Shift Arithmetic1 : ArithShift  BitShiftNumber=8  BitShiftDirection=Left
  Shift Arithmetic2 : ArithShift  BitShiftNumber=8  BitShiftDirection=Left
  Terminator{,1..3} (4 alike) : Terminator
  AMK_TempMotor : Outport
  AMK_TempInverter : Outport  Port=2
  wires:
  Data Type Conversion2/1 -> AMK_TempInverter/1
  Gain/1 -> Data Type Conversion1/1
  Add1/1 -> Gain/1
  Data Type Conversion1/1 -> AMK_TempMotor/1
  Data Type Conversion4/1 -> Add1/1
  Data Type Conversion5/1 -> Shift Arithmetic1/1
  Shift Arithmetic2/1 -> Add2/2
  Add2/1 -> Gain1/1
  Shift Arithmetic1/1 -> Add1/2
  Demux/2 -> Data Type Conversion5/1
  Gain1/1 -> Data Type Conversion2/1
  Demux/1 -> Data Type Conversion4/1
  Data Type Conversion3/1 -> Add2/1
  In1/1 -> Demux/1
  Data Type Conversion6/1 -> Shift Arithmetic2/1
  Demux/6 -> Terminator1/1
  Demux/5 -> Terminator/1
  Demux/4 -> Data Type Conversion6/1
  Demux/3 -> Data Type Conversion3/1
  Demux/8 -> Terminator3/1
  Demux/7 -> Terminator2/1

== system SS_1029/HardWare_Input/In3_Message/Function-Call Subsystem/Subsystem1 ==
  In1 : Inport
  Enable : EnablePort
  Add : Sum
  Add1 : Sum
  Data Type Conversion : DataTypeConversion  OutDataTypeStr=uint8
  Data Type Conversion{1..6} (6 alike) : DataTypeConversion  OutDataTypeStr=uint16
  Demux : Demux  Outputs=8
  Shift Arithmetic1 : ArithShift  BitShiftNumber=8  BitShiftDirection=Left
  Shift Arithmetic2 : ArithShift  BitShiftNumber=8  BitShiftDirection=Left
  Subsystem : Subsystem
  Terminator : Terminator
  Terminator1 : Terminator
  Terminator2 : Terminator
  Out1 : Outport
  Out2 : Outport  Port=2
  Out3 : Outport  Port=3
  Out4 : Outport  Port=4
  Out5 : Outport  Port=5
  Out6 : Outport  Port=6
  wires:
  In1/1 -> Demux/1
  Demux/1 -> Terminator/1
  Add1/1 -> Data Type Conversion6/1
  Data Type Conversion6/1 -> Out6/1
  Add/1 -> Data Type Conversion3/1
  Data Type Conversion/1 -> Subsystem/1(In1)
  Demux/3 -> Data Type Conversion1/1
  Demux/5 -> Data Type Conversion4/1
  Demux/6 -> Data Type Conversion5/1
  Demux/2 -> Data Type Conversion/1
  Demux/4 -> Data Type Conversion2/1
  Data Type Conversion2/1 -> Shift Arithmetic2/1
  Shift Arithmetic2/1 -> Add/2
  Data Type Conversion1/1 -> Add/1
  Data Type Conversion3/1 -> Out5/1
  Data Type Conversion5/1 -> Shift Arithmetic1/1
  Data Type Conversion4/1 -> Add1/1
  Shift Arithmetic1/1 -> Add1/2
  Subsystem/1(AMK_bSystemReady) -> Out1/1
  Subsystem/4(AMK_bQuitInverterOn) -> Out4/1
  Subsystem/3(AMK_bQuitDcOn) -> Out3/1
  Demux/7 -> Terminator1/1
  Subsystem/2(AMK_bError) -> Out2/1
  Demux/8 -> Terminator2/1

== system SS_1029/HardWare_Input/In3_Message/Function-Call Subsystem1/Subsystem ==
  In1 : Inport
  Enable : EnablePort
  Add1 : Sum
  Add2 : Sum
  Data Type Conversion1 : DataTypeConversion  OutDataTypeStr=single
  Data Type Conversion2 : DataTypeConversion  OutDataTypeStr=single
  Data Type Conversion{3..6} (4 alike) : DataTypeConversion  OutDataTypeStr=uint16
  Demux : Demux  Outputs=8
  Gain : Gain  Gain=0.1
  Gain1 : Gain  Gain=0.1
  Shift Arithmetic1 : ArithShift  BitShiftNumber=8  BitShiftDirection=Left
  Shift Arithmetic2 : ArithShift  BitShiftNumber=8  BitShiftDirection=Left
  Terminator{,1..3} (4 alike) : Terminator
  AMK_TempMotor : Outport
  AMK_TempInverter : Outport  Port=2
  wires:
  Data Type Conversion2/1 -> AMK_TempInverter/1
  Gain/1 -> Data Type Conversion1/1
  Add1/1 -> Gain/1
  Data Type Conversion1/1 -> AMK_TempMotor/1
  Data Type Conversion4/1 -> Add1/1
  Data Type Conversion5/1 -> Shift Arithmetic1/1
  Shift Arithmetic2/1 -> Add2/2
  Add2/1 -> Gain1/1
  Shift Arithmetic1/1 -> Add1/2
  Demux/2 -> Data Type Conversion5/1
  Gain1/1 -> Data Type Conversion2/1
  Demux/1 -> Data Type Conversion4/1
  Data Type Conversion3/1 -> Add2/1
  In1/1 -> Demux/1
  Data Type Conversion6/1 -> Shift Arithmetic2/1
  Demux/6 -> Terminator1/1
  Demux/5 -> Terminator/1
  Demux/4 -> Data Type Conversion6/1
  Demux/3 -> Data Type Conversion3/1
  Demux/8 -> Terminator3/1
  Demux/7 -> Terminator2/1

== system SS_1029/HardWare_Input/In4_Message/Function-Call Subsystem/Subsystem1 ==
  In1 : Inport
  Enable : EnablePort
  Add : Sum
  Add1 : Sum
  Data Type Conversion : DataTypeConversion  OutDataTypeStr=uint8
  Data Type Conversion{1..6} (6 alike) : DataTypeConversion  OutDataTypeStr=uint16
  Demux : Demux  Outputs=8
  Shift Arithmetic1 : ArithShift  BitShiftNumber=8  BitShiftDirection=Left
  Shift Arithmetic2 : ArithShift  BitShiftNumber=8  BitShiftDirection=Left
  Subsystem : Subsystem
  Terminator : Terminator
  Terminator1 : Terminator
  Terminator2 : Terminator
  Out1 : Outport
  Out2 : Outport  Port=2
  Out3 : Outport  Port=3
  Out4 : Outport  Port=4
  Out5 : Outport  Port=5
  Out6 : Outport  Port=6
  wires:
  In1/1 -> Demux/1
  Demux/1 -> Terminator/1
  Add1/1 -> Data Type Conversion6/1
  Data Type Conversion6/1 -> Out6/1
  Add/1 -> Data Type Conversion3/1
  Data Type Conversion/1 -> Subsystem/1(In1)
  Demux/3 -> Data Type Conversion1/1
  Demux/5 -> Data Type Conversion4/1
  Demux/6 -> Data Type Conversion5/1
  Demux/2 -> Data Type Conversion/1
  Demux/4 -> Data Type Conversion2/1
  Data Type Conversion2/1 -> Shift Arithmetic2/1
  Shift Arithmetic2/1 -> Add/2
  Data Type Conversion1/1 -> Add/1
  Data Type Conversion3/1 -> Out5/1
  Data Type Conversion5/1 -> Shift Arithmetic1/1
  Data Type Conversion4/1 -> Add1/1
  Shift Arithmetic1/1 -> Add1/2
  Subsystem/1(AMK_bSystemReady) -> Out1/1
  Subsystem/4(AMK_bQuitInverterOn) -> Out4/1
  Subsystem/3(AMK_bQuitDcOn) -> Out3/1
  Demux/7 -> Terminator1/1
  Subsystem/2(AMK_bError) -> Out2/1
  Demux/8 -> Terminator2/1

== system SS_1029/HardWare_Input/In4_Message/Function-Call Subsystem1/Subsystem ==
  In1 : Inport
  Enable : EnablePort
  Add1 : Sum
  Add2 : Sum
  Data Type Conversion1 : DataTypeConversion  OutDataTypeStr=single
  Data Type Conversion2 : DataTypeConversion  OutDataTypeStr=single
  Data Type Conversion{3..6} (4 alike) : DataTypeConversion  OutDataTypeStr=uint16
  Demux : Demux  Outputs=8
  Gain : Gain  Gain=0.1
  Gain1 : Gain  Gain=0.1
  Shift Arithmetic1 : ArithShift  BitShiftNumber=8  BitShiftDirection=Left
  Shift Arithmetic2 : ArithShift  BitShiftNumber=8  BitShiftDirection=Left
  Terminator{,1..3} (4 alike) : Terminator
  AMK_TempMotor : Outport
  AMK_TempInverter : Outport  Port=2
  wires:
  Data Type Conversion2/1 -> AMK_TempInverter/1
  Gain/1 -> Data Type Conversion1/1
  Add1/1 -> Gain/1
  Data Type Conversion1/1 -> AMK_TempMotor/1
  Data Type Conversion4/1 -> Add1/1
  Data Type Conversion5/1 -> Shift Arithmetic1/1
  Shift Arithmetic2/1 -> Add2/2
  Add2/1 -> Gain1/1
  Shift Arithmetic1/1 -> Add1/2
  Demux/2 -> Data Type Conversion5/1
  Gain1/1 -> Data Type Conversion2/1
  Demux/1 -> Data Type Conversion4/1
  Data Type Conversion3/1 -> Add2/1
  In1/1 -> Demux/1
  Data Type Conversion6/1 -> Shift Arithmetic2/1
  Demux/6 -> Terminator1/1
  Demux/5 -> Terminator/1
  Demux/4 -> Data Type Conversion6/1
  Demux/3 -> Data Type Conversion3/1
  Demux/8 -> Terminator3/1
  Demux/7 -> Terminator2/1

== system SS_1029/VCU_MCU/Enabled Subsystem/Atomic Subsystem4/Atomic Subsystem ==
  AMK_bErrorReset : Inport
  AMK_bEnable : Inport  Port=2
  AMK_bDcOn : Inport  Port=3
  AMK_bInverterOn : Inport  Port=4
  Add : Sum  Inputs=++++
  Bitwise Operator{,1..3} (4 alike) : simulink/Logic and Bit Operations/Bitwise Operator  logicop=AND  UseBitMask=on  BitMask=bin2dec('00000001')  BitMaskRealWorld=Stored Integer
  Bitwise Operator4 : simulink/Logic and Bit Operations/Bitwise Operator  logicop=AND  UseBitMask=on  BitMask=bin2dec('00001000')  BitMaskRealWorld=Stored Integer
  Bitwise Operator5 : simulink/Logic and Bit Operations/Bitwise Operator  logicop=AND  UseBitMask=on  BitMask=bin2dec('00000100')  BitMaskRealWorld=Stored Integer
  Bitwise Operator6 : simulink/Logic and Bit Operations/Bitwise Operator  logicop=AND  UseBitMask=on  BitMask=bin2dec('00000010')  BitMaskRealWorld=Stored Integer
  Shift Arithmetic1 : ArithShift  BitShiftNumber=2  BitShiftDirection=Left
  Shift Arithmetic2 : ArithShift  BitShiftNumber=3  BitShiftDirection=Left
  Shift Arithmetic3 : ArithShift  BitShiftNumber=1  BitShiftDirection=Left
  Out1 : Outport
  wires:
  AMK_bErrorReset/1 -> Bitwise Operator/1
  AMK_bEnable/1 -> Bitwise Operator1/1
  AMK_bDcOn/1 -> Bitwise Operator2/1
  AMK_bInverterOn/1 -> Bitwise Operator3/1
  Add/1 -> Out1/1
  Bitwise Operator3/1 -> Add/4
  Bitwise Operator/1 -> Shift Arithmetic2/1
  Bitwise Operator1/1 -> Shift Arithmetic1/1
  Bitwise Operator2/1 -> Shift Arithmetic3/1
  Shift Arithmetic3/1 -> Bitwise Operator6/1
  Shift Arithmetic1/1 -> Bitwise Operator5/1
  Shift Arithmetic2/1 -> Bitwise Operator4/1
  Bitwise Operator4/1 -> Add/1
  Bitwise Operator5/1 -> Add/2
  Bitwise Operator6/1 -> Add/3

== system SS_1029/VCU_MCU/Enabled Subsystem/Atomic Subsystem5/Atomic Subsystem ==
  AMK_bErrorReset : Inport
  AMK_bEnable : Inport  Port=2
  AMK_bDcOn : Inport  Port=3
  AMK_bInverterOn : Inport  Port=4
  Add : Sum  Inputs=++++
  Bitwise Operator{,1..3} (4 alike) : simulink/Logic and Bit Operations/Bitwise Operator  logicop=AND  UseBitMask=on  BitMask=bin2dec('00000001')  BitMaskRealWorld=Stored Integer
  Bitwise Operator4 : simulink/Logic and Bit Operations/Bitwise Operator  logicop=AND  UseBitMask=on  BitMask=bin2dec('00001000')  BitMaskRealWorld=Stored Integer
  Bitwise Operator5 : simulink/Logic and Bit Operations/Bitwise Operator  logicop=AND  UseBitMask=on  BitMask=bin2dec('00000100')  BitMaskRealWorld=Stored Integer
  Bitwise Operator6 : simulink/Logic and Bit Operations/Bitwise Operator  logicop=AND  UseBitMask=on  BitMask=bin2dec('00000010')  BitMaskRealWorld=Stored Integer
  Shift Arithmetic1 : ArithShift  BitShiftNumber=2  BitShiftDirection=Left
  Shift Arithmetic2 : ArithShift  BitShiftNumber=3  BitShiftDirection=Left
  Shift Arithmetic3 : ArithShift  BitShiftNumber=1  BitShiftDirection=Left
  Out1 : Outport
  wires:
  AMK_bErrorReset/1 -> Bitwise Operator/1
  AMK_bEnable/1 -> Bitwise Operator1/1
  AMK_bDcOn/1 -> Bitwise Operator2/1
  AMK_bInverterOn/1 -> Bitwise Operator3/1
  Add/1 -> Out1/1
  Bitwise Operator3/1 -> Add/4
  Bitwise Operator/1 -> Shift Arithmetic2/1
  Bitwise Operator1/1 -> Shift Arithmetic1/1
  Bitwise Operator2/1 -> Shift Arithmetic3/1
  Shift Arithmetic3/1 -> Bitwise Operator6/1
  Shift Arithmetic1/1 -> Bitwise Operator5/1
  Shift Arithmetic2/1 -> Bitwise Operator4/1
  Bitwise Operator4/1 -> Add/1
  Bitwise Operator5/1 -> Add/2
  Bitwise Operator6/1 -> Add/3

== system SS_1029/VCU_MCU/Enabled Subsystem/Atomic Subsystem6/Atomic Subsystem ==
  AMK_bErrorReset : Inport
  AMK_bEnable : Inport  Port=2
  AMK_bDcOn : Inport  Port=3
  AMK_bInverterOn : Inport  Port=4
  Add : Sum  Inputs=++++
  Bitwise Operator{,1..3} (4 alike) : simulink/Logic and Bit Operations/Bitwise Operator  logicop=AND  UseBitMask=on  BitMask=bin2dec('00000001')  BitMaskRealWorld=Stored Integer
  Bitwise Operator4 : simulink/Logic and Bit Operations/Bitwise Operator  logicop=AND  UseBitMask=on  BitMask=bin2dec('00001000')  BitMaskRealWorld=Stored Integer
  Bitwise Operator5 : simulink/Logic and Bit Operations/Bitwise Operator  logicop=AND  UseBitMask=on  BitMask=bin2dec('00000100')  BitMaskRealWorld=Stored Integer
  Bitwise Operator6 : simulink/Logic and Bit Operations/Bitwise Operator  logicop=AND  UseBitMask=on  BitMask=bin2dec('00000010')  BitMaskRealWorld=Stored Integer
  Shift Arithmetic1 : ArithShift  BitShiftNumber=2  BitShiftDirection=Left
  Shift Arithmetic2 : ArithShift  BitShiftNumber=3  BitShiftDirection=Left
  Shift Arithmetic3 : ArithShift  BitShiftNumber=1  BitShiftDirection=Left
  Out1 : Outport
  wires:
  AMK_bErrorReset/1 -> Bitwise Operator/1
  AMK_bEnable/1 -> Bitwise Operator1/1
  AMK_bDcOn/1 -> Bitwise Operator2/1
  AMK_bInverterOn/1 -> Bitwise Operator3/1
  Add/1 -> Out1/1
  Bitwise Operator3/1 -> Add/4
  Bitwise Operator/1 -> Shift Arithmetic2/1
  Bitwise Operator1/1 -> Shift Arithmetic1/1
  Bitwise Operator2/1 -> Shift Arithmetic3/1
  Shift Arithmetic3/1 -> Bitwise Operator6/1
  Shift Arithmetic1/1 -> Bitwise Operator5/1
  Shift Arithmetic2/1 -> Bitwise Operator4/1
  Bitwise Operator4/1 -> Add/1
  Bitwise Operator5/1 -> Add/2
  Bitwise Operator6/1 -> Add/3

== system SS_1029/VCU_MCU/Enabled Subsystem/Atomic Subsystem7/Atomic Subsystem ==
  AMK_bErrorReset : Inport
  AMK_bEnable : Inport  Port=2
  AMK_bDcOn : Inport  Port=3
  AMK_bInverterOn : Inport  Port=4
  Add : Sum  Inputs=++++
  Bitwise Operator{,1..3} (4 alike) : simulink/Logic and Bit Operations/Bitwise Operator  logicop=AND  UseBitMask=on  BitMask=bin2dec('00000001')  BitMaskRealWorld=Stored Integer
  Bitwise Operator4 : simulink/Logic and Bit Operations/Bitwise Operator  logicop=AND  UseBitMask=on  BitMask=bin2dec('00001000')  BitMaskRealWorld=Stored Integer
  Bitwise Operator5 : simulink/Logic and Bit Operations/Bitwise Operator  logicop=AND  UseBitMask=on  BitMask=bin2dec('00000100')  BitMaskRealWorld=Stored Integer
  Bitwise Operator6 : simulink/Logic and Bit Operations/Bitwise Operator  logicop=AND  UseBitMask=on  BitMask=bin2dec('00000010')  BitMaskRealWorld=Stored Integer
  Shift Arithmetic1 : ArithShift  BitShiftNumber=2  BitShiftDirection=Left
  Shift Arithmetic2 : ArithShift  BitShiftNumber=3  BitShiftDirection=Left
  Shift Arithmetic3 : ArithShift  BitShiftNumber=1  BitShiftDirection=Left
  Out1 : Outport
  wires:
  AMK_bErrorReset/1 -> Bitwise Operator/1
  AMK_bEnable/1 -> Bitwise Operator1/1
  AMK_bDcOn/1 -> Bitwise Operator2/1
  AMK_bInverterOn/1 -> Bitwise Operator3/1
  Add/1 -> Out1/1
  Bitwise Operator3/1 -> Add/4
  Bitwise Operator/1 -> Shift Arithmetic2/1
  Bitwise Operator1/1 -> Shift Arithmetic1/1
  Bitwise Operator2/1 -> Shift Arithmetic3/1
  Shift Arithmetic3/1 -> Bitwise Operator6/1
  Shift Arithmetic1/1 -> Bitwise Operator5/1
  Shift Arithmetic2/1 -> Bitwise Operator4/1
  Bitwise Operator4/1 -> Add/1
  Bitwise Operator5/1 -> Add/2
  Bitwise Operator6/1 -> Add/3

== system SS_1029/VCU_MCU/Enabled Subsystem/Torquearrengement/AMK1 ==
  v : Inport
  Taim : Inport  Port=2
  1-D Lookup Table : Lookup_n-D  NumberOfTableDimensions=1  BreakpointsForDimension1=[0 13000 14000 15000 16000 17000 18000 19000]  Table=[21 21 20 17 16 13 8 0]  ExtrapMethod=Clip  InternalRulePriority=Speed  RndMeth=Simplest  InputSameDT=on
  Constant : Constant  Value=0.0098  SampleTime=-1
  Divide : Product  Inputs=*/  OutDataTypeStr=single
  Divide1 : Product  Inputs=*/  OutDataTypeStr=single
  Saturation : Saturate  UpperLimit=2000  LowerLimit=0
  "ReduceFactor " : Outport
  wires:
  v/1 -> 1-D Lookup Table/1
  1-D Lookup Table/1 -> Divide/1
  Constant/1 -> Divide/2
  Divide/1 -> Saturation/1
  Taim/1 -> Divide1/2
  Divide1/1 -> "ReduceFactor "/1
  Saturation/1 -> Divide1/1

== system SS_1029/VCU_MCU/Enabled Subsystem/Torquearrengement/AMK2 ==
  v : Inport
  Taim : Inport  Port=2
  1-D Lookup Table : Lookup_n-D  NumberOfTableDimensions=1  BreakpointsForDimension1=[0 13000 14000 15000 16000 17000 18000 19000]  Table=[21 21 20 17 16 13 8 0]  ExtrapMethod=Clip  InternalRulePriority=Speed  RndMeth=Simplest  InputSameDT=on
  Constant : Constant  Value=0.0098  SampleTime=-1
  Divide : Product  Inputs=*/  OutDataTypeStr=single
  Divide1 : Product  Inputs=*/  OutDataTypeStr=single
  Saturation : Saturate  UpperLimit=2000  LowerLimit=0
  "ReduceFactor " : Outport
  wires:
  v/1 -> 1-D Lookup Table/1
  1-D Lookup Table/1 -> Divide/1
  Constant/1 -> Divide/2
  Divide/1 -> Saturation/1
  Taim/1 -> Divide1/2
  Divide1/1 -> "ReduceFactor "/1
  Saturation/1 -> Divide1/1

== system SS_1029/VCU_MCU/Enabled Subsystem/Torquearrengement/AMK3 ==
  v : Inport
  Taim : Inport  Port=2
  1-D Lookup Table : Lookup_n-D  NumberOfTableDimensions=1  BreakpointsForDimension1=[0 13000 14000 15000 16000 17000 18000 19000]  Table=[21 21 20 17 16 13 8 0]  ExtrapMethod=Clip  InternalRulePriority=Speed  RndMeth=Simplest  InputSameDT=on
  Constant : Constant  Value=0.0098  SampleTime=-1
  Divide : Product  Inputs=*/  OutDataTypeStr=single
  Divide1 : Product  Inputs=*/  OutDataTypeStr=single
  Saturation : Saturate  UpperLimit=2000  LowerLimit=0
  "ReduceFactor " : Outport
  wires:
  v/1 -> 1-D Lookup Table/1
  1-D Lookup Table/1 -> Divide/1
  Constant/1 -> Divide/2
  Divide/1 -> Saturation/1
  Taim/1 -> Divide1/2
  Divide1/1 -> "ReduceFactor "/1
  Saturation/1 -> Divide1/1

== system SS_1029/VCU_MCU/Enabled Subsystem/Torquearrengement/AMK4 ==
  v : Inport
  Taim : Inport  Port=2
  1-D Lookup Table : Lookup_n-D  NumberOfTableDimensions=1  BreakpointsForDimension1=[0 13000 14000 15000 16000 17000 18000 19000]  Table=[21 21 20 17 16 13 8 0]  ExtrapMethod=Clip  InternalRulePriority=Speed  RndMeth=Simplest  InputSameDT=on
  Constant : Constant  Value=0.0098  SampleTime=-1
  Divide : Product  Inputs=*/  OutDataTypeStr=single
  Divide1 : Product  Inputs=*/  OutDataTypeStr=single
  Saturation : Saturate  UpperLimit=2000  LowerLimit=0
  "ReduceFactor " : Outport
  wires:
  v/1 -> 1-D Lookup Table/1
  1-D Lookup Table/1 -> Divide/1
  Constant/1 -> Divide/2
  Divide/1 -> Saturation/1
  Taim/1 -> Divide1/2
  Divide1/1 -> "ReduceFactor "/1
  Saturation/1 -> Divide1/1
